simulink model "B737_CAS"  (R2018a)
settings: Solver=VariableStepAuto  StartTime=0.0  StopTime=S.simtime  RelTol=1e-3
undefined symbols (not defined in the file): S, sigbuilder_block
settings Model: Creator=Can Bekar  LastModifiedBy=Can Bekar
settings DataIOCC: ExternalInput=S.usignal  LoadExternalInput=on  SignalLogging=off  DSMLogging=off

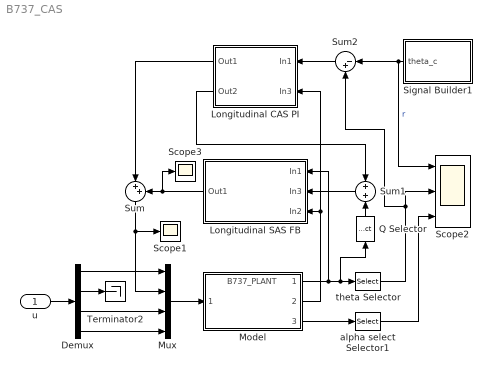
== system B737_CAS ==
  u : Inport
  Demux : Demux
  Longitudinal CAS PI : Subsystem
  Longitudinal SAS FB : Subsystem
  Model : ModelReference  ModelNameDialog=B737_PLANT  SimulationMode=Normal  ModelReferenceVersion=1.6
  Mux : Mux
  Q Selector : Selector  InputPortWidth=12  IndexOptions=Index vector (dialog)  Indices=[8]  OutputSizes=1
  Scope1 : Scope
  Scope2 : Scope  NumInputPorts=3
  Scope3 : Scope
  Signal Builder1 : Subsystem  Tag=STV Subsys  LoadFcn=sigbuilder_block('load');  StartFcn=sigbuilder_block('start');  StopFcn=sigbuilder_block('stop');  ClipboardFcn=sigbuilder_block('clipboard');  mask(Sigbuilder block){tuvar=[0:10]}
      mask help: Simulink:masks:SigbuilderBlock_MD
      mask init:
      | if ~strcmp(get_param(bdroot(gcbh),'SimulationStatus'),'stopped') tuvar = sigbuilder_block('maskInit'); end
      settings: CopyFcn=sigbuilder_block('copy');  DeleteFcn=sigbuilder_block('delete');  ModelCloseFcn=sigbuilder_block('modelClose');  PreSaveFcn=sigbuilder_block('preSave');  PauseFcn=sigbuilder_block('pause');  ContinueFcn=sigbuilder_block('continue');  NameChangeFcn=sigbuilder_block('namechange');  OpenFcn=sigbuilder_block('open',[233.25 91.5 964.5 399.75 ]);  CloseFcn=sigbuilder_block('close');
      mask Display: plot(0, 0, 100, 100,[2, 2, 32, 32, 2], [68, 8, 8, 68, 68],[32, 2], [38, 38], [32, 19, 2],[53, 60, 44], [32, 17, 17, 2],[16, 16, 31, 31]);txt = getActiveGroup(gcbh);text(2, 100, txt,'verticalAlignment', 'top');
  Sum : Sum  Inputs=|++
  Sum1 : Sum  Inputs=+|+
  Sum2 : Sum  Inputs=|-+
  Terminator2 : Terminator
  alpha select Selector1 : Selector  InputPortWidth=12  IndexOptions=Index vector (dialog)  Indices=[12]  OutputSizes=1
  theta Selector : Selector  InputPortWidth=12  IndexOptions=Index vector (dialog)  Indices=[5]  OutputSizes=1
  wires:
  u/1 -> Demux/1
  Mux/1 -> Model/1
  Demux/1 -> Mux/1
  Demux/3 -> Mux/3
  Demux/4 -> Mux/4
  Sum/1 -> Mux/2, Scope1/1
  Demux/2 -> Terminator2/1
  Signal Builder1/1(theta_c) -> Sum2/1, Scope2/1  "r"
  Model/2 -> Longitudinal CAS PI/2(In3), Longitudinal SAS FB/3(In2)
  Longitudinal SAS FB/1(Out1) -> Scope3/1, Sum/2
  Longitudinal CAS PI/1(Out1) -> Sum/1
  Longitudinal CAS PI/2(Out2) -> Sum1/1
  Q Selector/1 -> Sum1/2
  Model/1 -> Longitudinal SAS FB/1(In1), Q Selector/1, theta Selector/1
  theta Selector/1 -> Sum2/2, Scope2/2
  Sum1/1 -> Longitudinal SAS FB/2(In3)
  Sum2/1 -> Longitudinal CAS PI/1(In1)
  Model/3 -> alpha select Selector1/1
  alpha select Selector1/1 -> Scope2/3

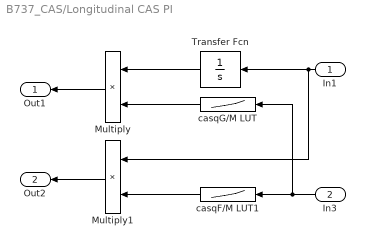
== system B737_CAS/Longitudinal CAS PI ==
  In1 : Inport
  In3 : Inport  Port=2
  Multiply : Product
  Multiply1 : Product
  Transfer Fcn : TransferFcn  Denominator=[1 0]
  casqF/M LUT1 : Lookup_n-D  NumberOfTableDimensions=1  BreakpointsForDimension1=S.M'  Table=S.casqFLUT  InternalRulePriority=Speed  RndMeth=Simplest  InputSameDT=on
  casqG/M LUT : Lookup_n-D  NumberOfTableDimensions=1  BreakpointsForDimension1=S.M'  Table=S.casqGLUT  InternalRulePriority=Speed  RndMeth=Simplest  InputSameDT=on
  Out1 : Outport
  Out2 : Outport  Port=2
  wires:
  Multiply/1 -> Out1/1
  casqG/M LUT/1 -> Multiply/2
  casqF/M LUT1/1 -> Multiply1/2
  In3/1 -> casqG/M LUT/1, casqF/M LUT1/1
  Multiply1/1 -> Out2/1
  In1/1 -> Multiply1/1, Transfer Fcn/1
  Transfer Fcn/1 -> Multiply/1

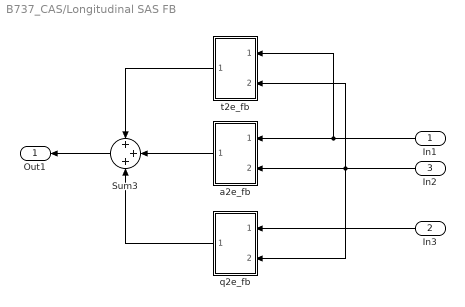
== system B737_CAS/Longitudinal SAS FB ==
  In1 : Inport
  In3 : Inport  Port=2
  In2 : Inport  Port=3
  Sum3 : Sum  Inputs=+++
  a2e_fb : Subsystem
  q2e_fb : Subsystem
  t2e_fb : Subsystem
  Out1 : Outport
  wires:
  Sum3/1 -> Out1/1
  In2/1 -> q2e_fb/2(In2), a2e_fb/2(In2), t2e_fb/2(In2)
  In1/1 -> a2e_fb/1(In1), t2e_fb/1(In1)
  q2e_fb/1(Out1) -> Sum3/3
  t2e_fb/1(Out1) -> Sum3/1
  a2e_fb/1(Out1) -> Sum3/2
  In3/1 -> q2e_fb/1(In3)

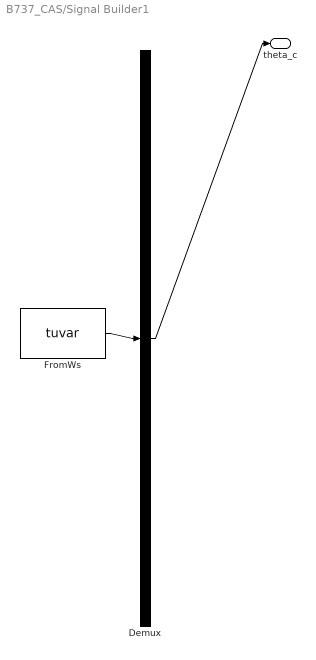
== system B737_CAS/Signal Builder1 ==
  Demux : Demux  Tag=STV Demux  Outputs=1
  FromWs : FromWorkspace  Tag=STV FromWs  VariableName=tuvar  SampleTime=0
      SigBuilderData=|
      | common.afterFinalStr = 'Extrapolate'
      | common.sampleTime = 0
      | dataSet.timeRange = [0 300]
      | dataSet.name = 'Group 1'
      | sbobj.Groups.Name = 'Group 1'
      | sbobj.Groups.Signals.Name = 'theta_c'
      | sbobj.Groups.Signals.XData = [0 50 50 100 100 150.5 150.5 201 250.5 250.5 300]
      | sbobj.Groups.Signals.YData = [-5e-05 -5e-05 0.00345 0.00345 -5e-05 0.0029 -0.0033 -0.0061 -0.0002 -5e-05 -5e-05]
      | sbobj.Groups.TimeRange = [0 300]
  theta_c : Outport  Tag=STV Outport
  wires:
  Demux/1 -> theta_c/1
  FromWs/1 -> Demux/1

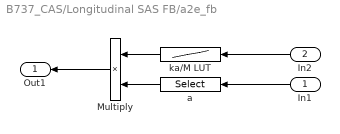
== system B737_CAS/Longitudinal SAS FB/a2e_fb ==
  In1 : Inport
  In2 : Inport  Port=2
  Multiply : Product
  a : Selector  InputPortWidth=12  IndexOptions=Index vector (dialog)  Indices=[2]  OutputSizes=1
  ka/M LUT : Lookup_n-D  NumberOfTableDimensions=1  BreakpointsForDimension1=S.M'  Table=S.kaLUT2  InternalRulePriority=Speed  RndMeth=Simplest  InputSameDT=on
  Out1 : Outport
  wires:
  Multiply/1 -> Out1/1
  ka/M LUT/1 -> Multiply/1
  In2/1 -> ka/M LUT/1
  In1/1 -> a/1
  a/1 -> Multiply/2

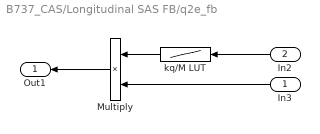
== system B737_CAS/Longitudinal SAS FB/q2e_fb ==
  In3 : Inport
  In2 : Inport  Port=2
  Multiply : Product
  kq/M LUT : Lookup_n-D  NumberOfTableDimensions=1  BreakpointsForDimension1=S.M'  Table=S.kqLUT2  InternalRulePriority=Speed  RndMeth=Simplest  InputSameDT=on
  Out1 : Outport
  wires:
  In2/1 -> kq/M LUT/1
  kq/M LUT/1 -> Multiply/1
  Multiply/1 -> Out1/1
  In3/1 -> Multiply/2

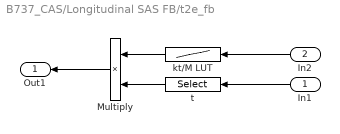
== system B737_CAS/Longitudinal SAS FB/t2e_fb ==
  In1 : Inport
  In2 : Inport  Port=2
  Multiply : Product
  kt/M LUT : Lookup_n-D  NumberOfTableDimensions=1  BreakpointsForDimension1=S.M'  Table=S.ktLUT2  InternalRulePriority=Speed  RndMeth=Simplest  InputSameDT=on
  t : Selector  InputPortWidth=12  IndexOptions=Index vector (dialog)  Indices=[5]  OutputSizes=1
  Out1 : Outport
  wires:
  t/1 -> Multiply/2
  In1/1 -> t/1
  In2/1 -> kt/M LUT/1
  kt/M LUT/1 -> Multiply/1
  Multiply/1 -> Out1/1
